simulink model "lorenz3d"  (Simulink 3.00)
settings: Solver=ode45  SolverMode=SingleTasking  StartTime=0.0  StopTime=inf  RelTol=1e-3  AbsTol=1e-6
undefined symbols (not defined in the file or in its folder): sfunxyz
settings Model: ExternalInput=[]  SaveTime=off  SaveOutput=off  InitialState=[]  IntegerOverflowMsg=none  RTWOptions="-aEnforceIntegerDowncast=1 -aFoldNonRolledExpr=1 -aInlineInvariantSignals=1 -aInlineParameters=0 -aLocalBlockOutputs=1 -aRollThreshold=5 -aZeroInternalMemoryAtStartup=1 -aZeroExternalMemoryAtStartup=1 -aInitFltsAndDblsToZero=1 -aGenerateReport=0 -aGenCodeOnly=0 -aRTWVerbose=1 -aIncludeHyperlinkInReport=0 -aLaunchReport=0 -aForceParamTrailComments=0 -aGenerateComments=1 -aIgnoreCustomStorageClasses=1 -aIncHierarchyInIds=0 -aMaxRTWIdLen=31 -aShowEliminatedStatements=0 -aPrefixModelToSubsysFcnNames=1 -aIncDataTypeInIds=0 -aInsertBlockDesc=0 -aSimulinkBlockComments=1 -aInlinedPrmAccess=\"Literals\"  -aSuppressErrorStatus=0 -aModelReferenceCompliant=1 -aSupportNonInlinedSFcns=1 -aSupportContinuousTime=1 -aSupportComplex=1 -aSupportNonFinite=1 -aSupportAbsoluteTime=1 -aTargetFcnLib=\"ansi_tfl_tmw.mat\" -aMultiInstanceERTCode=0 -aLogVarNameModifier=\"rt_\" -aIsPILTarget=0 -aCombineOutputUpdateFcns=0 -aGenerateASAP2=0 -aGenerateSampleERTMain=0 -aGenerateFullHeader=1 -aUtilityFuncGeneration=\"Auto\" -aIncludeFileDelimiter=\"Auto\" -aIncludeMdlTerminateFcn=1 -aPurelyIntegerCode=0 -aERTCustomFileBanners=0 -aRTWCAPIStates=0 -aRTWCAPIParams=0 -aRTWCAPISignals=0 -aMatFileLogging=1 -aGenFloatMathFcnCalls=\"ANSI_C\" -aExtModeMexFile=\"ext_comm\" -aExtModeTransport=0 -aExtModeStaticAllocSize=1000000 -aExtModeTesting=0 -aExtModeStaticAlloc=0 -aExtMode=0  -aInitFltsAndDblsToZero=1"  Creator=The MathWorks Inc.  LastModifiedBy=campa

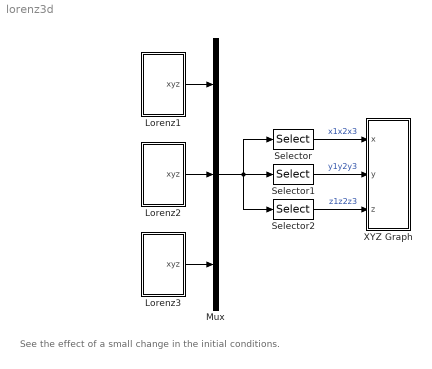
== system lorenz3d ==
  note: See the effect of a small change in the initial conditions.
  Lorenz1 : Subsystem  mask(Lorenz Attractor System){s=10, r=28, b=2+2/3, xyz0=[1 1 1]}
      mask prompts: s "sigma"; r "rho"; b "beta"; xyz0 "Initial State (x0, y0, y0)"
      mask help:
      | This autonomous system generates the lorentz attractor:
      | xdot=sigma*(x-y); ydot=rho*x-y-x*z; zdot=-beta*z+x*y;
      | Parameters and initial state can be selected from the mask.
      mask Help:
      | This autonomous system generates the lorentz attractor.
      | Parameters and initial state can be selected from the mask.
      | <p>
      | The system equations are:
      | xdot = sigma*(x-y),
      | ydot = rho*x-y-x*z,
      | zdot = -beta*z+x*y,
  Lorenz2 : Subsystem  mask(Lorenz Attractor System){s=10, r=28, b=2+2/3, xyz0=[2 2 2]}
      mask prompts: s "sigma"; r "rho"; b "beta"; xyz0 "Initial State (x0, y0, y0)"
      mask help:
      | This autonomous system generates the lorentz attractor:
      | xdot=sigma*(x-y); ydot=rho*x-y-x*z; zdot=-beta*z+x*y;
      | Parameters and initial state can be selected from the mask.
      mask Help:
      | This autonomous system generates the lorentz attractor.
      | Parameters and initial state can be selected from the mask.
      | <p>
      | The system equations are:
      | xdot = sigma*(x-y),
      | ydot = rho*x-y-x*z,
      | zdot = -beta*z+x*y,
  Lorenz3 : Subsystem  mask(Lorenz Attractor System){s=10, r=28, b=2+2/3, xyz0=[3 3 3]}
      mask prompts: s "sigma"; r "rho"; b "beta"; xyz0 "Initial State (x0, y0, y0)"
      mask help:
      | This autonomous system generates the lorentz attractor:
      | xdot=sigma*(x-y); ydot=rho*x-y-x*z; zdot=-beta*z+x*y;
      | Parameters and initial state can be selected from the mask.
      mask Help:
      | This autonomous system generates the lorentz attractor.
      | Parameters and initial state can be selected from the mask.
      | <p>
      | The system equations are:
      | xdot = sigma*(x-y),
      | ydot = rho*x-y-x*z,
      | zdot = -beta*z+x*y,
  Mux : Mux  Inputs=[3 3 3]
  Selector : Selector  Elements=[1 4 7]  InputPortWidth=9
  Selector1 : Selector  Elements=[2 5 8]  InputPortWidth=9
  Selector2 : Selector  Elements=[3 6 9]  InputPortWidth=9
  XYZ Graph : Subsystem  LoadFcn=sfunxyz([],[],[],'LoadBlock')  StartFcn=sfunxyz([],[],[],'Start')  StopFcn=sfunxyz([],[],[],'Stop')  mask(XYZ multiscope){np=3, xlim=[-30 30], ylim=[-20 30], zlim=[0 50], cp=[1 1 20], gd=on, st=0.01}
      mask prompts: np "Number of lines"; xlim "[xmin xmax]"; ylim "[ymin ymax]"; zlim "[zmin zmax]"; cp "Camera position (use [0 0 1] for 2D XY view)"; gd "Grid"; st "Sample time:"
      mask help:
      | Multidimensional XYZ scope using MATLAB graph window.
      |    X,Y,Z coordinates are respectively the first,second, and third input.
      |    Enter the number of lines, the XYZ ranges, the camera position,
      |    and the sampling time, as mask parameters.
      settings: CopyFcn=sfunxyz([],[],[],'CopyBlock')  DeleteFcn=sfunxyz([],[],[],'DeleteBlock')  NameChangeFcn=sfunxyz([],[],[],'NameChange')
      mask Help:
      | This block can be used to explore limit cycles.
      |    Look at the m-file sfunxyz.m to see how it works.
      mask Display: plot([.05 .95 .95 .05 .05],[.45 .45 .95 .95 .45], 0.5+cos(0:0.1:2*pi)*0.3,0.7+sin(0:0.1:2*pi)*0.2)
  wires:
  Lorenz1/1(xyz) -> Mux/1
  Lorenz2/1(xyz) -> Mux/2
  Mux/1 -> Selector/1, Selector1/1, Selector2/1
  Lorenz3/1(xyz) -> Mux/3
  Selector/1 -> XYZ Graph/1(x)  "x1x2x3"
  Selector1/1 -> XYZ Graph/2(y)  "y1y2y3"
  Selector2/1 -> XYZ Graph/3(z)  "z1z2z3"

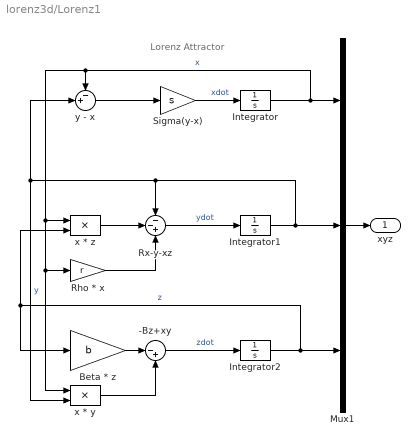
== system lorenz3d/Lorenz1 ==
  note: Lorenz Attractor
  -Bz+xy : Sum  Inputs=|-+  SaturateOnIntegerOverflow=on
  Beta * z : Gain  Gain=b  SaturateOnIntegerOverflow=on
  Integrator : Integrator  ExternalReset=none  InitialConditionSource=internal  InitialCondition=xyz0(1)  LimitOutput=off  UpperSaturationLimit=inf  LowerSaturationLimit=-inf  ShowSaturationPort=off  ShowStatePort=off  AbsoluteTolerance=auto
  Integrator1 : Integrator  ExternalReset=none  InitialConditionSource=internal  InitialCondition=xyz0(2)  LimitOutput=off  UpperSaturationLimit=inf  LowerSaturationLimit=-inf  ShowSaturationPort=off  ShowStatePort=off  AbsoluteTolerance=auto
  Integrator2 : Integrator  ExternalReset=none  InitialConditionSource=internal  InitialCondition=xyz0(3)  LimitOutput=off  UpperSaturationLimit=inf  LowerSaturationLimit=-inf  ShowSaturationPort=off  ShowStatePort=off  AbsoluteTolerance=auto
  Mux1 : Mux  Inputs=3
  Rho * x : Gain  Gain=r  SaturateOnIntegerOverflow=on
  Rx-y-xz : Sum  Inputs=--+  SaturateOnIntegerOverflow=on
  Sigma(y-x) : Gain  Gain=s  SaturateOnIntegerOverflow=on
  x * y : Product  Inputs=2  SaturateOnIntegerOverflow=on
  x * z : Product  Inputs=2  SaturateOnIntegerOverflow=on
  y - x : Sum  Inputs=-+|  SaturateOnIntegerOverflow=on
  xyz : Outport  Port=1
  wires:
  Sigma(y-x)/1 -> Integrator/1  "xdot"
  y - x/1 -> Sigma(y-x)/1
  Rx-y-xz/1 -> Integrator1/1  "ydot"
  x * z/1 -> Rx-y-xz/2
  Integrator2/1 -> x * z/2, Beta * z/1, Mux1/3  "z"
  Integrator1/1 -> Rx-y-xz/1, y - x/2, x * y/2, Mux1/2  "y"
  Integrator/1 -> y - x/1, x * z/1, Rho * x/1, x * y/1, Mux1/1  "x"
  -Bz+xy/1 -> Integrator2/1  "zdot"
  Beta * z/1 -> -Bz+xy/1
  x * y/1 -> -Bz+xy/2
  Mux1/1 -> xyz/1
  Rho * x/1 -> Rx-y-xz/3

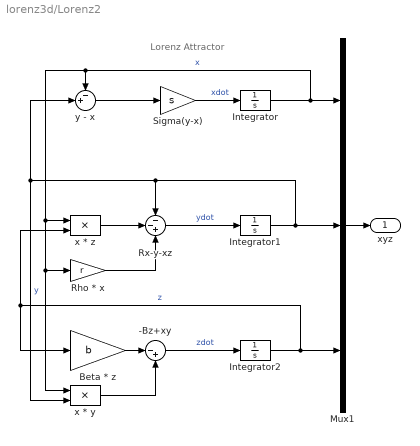
== system lorenz3d/Lorenz2 ==
  note: Lorenz Attractor
  -Bz+xy : Sum  Inputs=|-+  SaturateOnIntegerOverflow=on
  Beta * z : Gain  Gain=b  SaturateOnIntegerOverflow=on
  Integrator : Integrator  ExternalReset=none  InitialConditionSource=internal  InitialCondition=xyz0(1)  LimitOutput=off  UpperSaturationLimit=inf  LowerSaturationLimit=-inf  ShowSaturationPort=off  ShowStatePort=off  AbsoluteTolerance=auto
  Integrator1 : Integrator  ExternalReset=none  InitialConditionSource=internal  InitialCondition=xyz0(2)  LimitOutput=off  UpperSaturationLimit=inf  LowerSaturationLimit=-inf  ShowSaturationPort=off  ShowStatePort=off  AbsoluteTolerance=auto
  Integrator2 : Integrator  ExternalReset=none  InitialConditionSource=internal  InitialCondition=xyz0(3)  LimitOutput=off  UpperSaturationLimit=inf  LowerSaturationLimit=-inf  ShowSaturationPort=off  ShowStatePort=off  AbsoluteTolerance=auto
  Mux1 : Mux  Inputs=3
  Rho * x : Gain  Gain=r  SaturateOnIntegerOverflow=on
  Rx-y-xz : Sum  Inputs=--+  SaturateOnIntegerOverflow=on
  Sigma(y-x) : Gain  Gain=s  SaturateOnIntegerOverflow=on
  x * y : Product  Inputs=2  SaturateOnIntegerOverflow=on
  x * z : Product  Inputs=2  SaturateOnIntegerOverflow=on
  y - x : Sum  Inputs=-+|  SaturateOnIntegerOverflow=on
  xyz : Outport  Port=1
  wires:
  Mux1/1 -> xyz/1
  x * y/1 -> -Bz+xy/2
  Beta * z/1 -> -Bz+xy/1
  -Bz+xy/1 -> Integrator2/1  "zdot"
  Integrator/1 -> Mux1/1, x * y/1, Rho * x/1, x * z/1, y - x/1  "x"
  Integrator1/1 -> Mux1/2, x * y/2, y - x/2, Rx-y-xz/1  "y"
  Integrator2/1 -> Mux1/3, Beta * z/1, x * z/2  "z"
  x * z/1 -> Rx-y-xz/2
  Rx-y-xz/1 -> Integrator1/1  "ydot"
  y - x/1 -> Sigma(y-x)/1
  Sigma(y-x)/1 -> Integrator/1  "xdot"
  Rho * x/1 -> Rx-y-xz/3

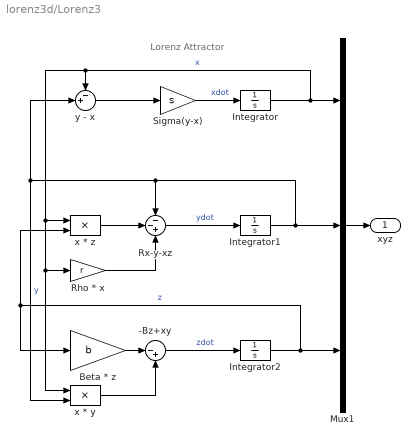
== system lorenz3d/Lorenz3 ==
  note: Lorenz Attractor
  -Bz+xy : Sum  Inputs=|-+  SaturateOnIntegerOverflow=on
  Beta * z : Gain  Gain=b  SaturateOnIntegerOverflow=on
  Integrator : Integrator  ExternalReset=none  InitialConditionSource=internal  InitialCondition=xyz0(1)  LimitOutput=off  UpperSaturationLimit=inf  LowerSaturationLimit=-inf  ShowSaturationPort=off  ShowStatePort=off  AbsoluteTolerance=auto
  Integrator1 : Integrator  ExternalReset=none  InitialConditionSource=internal  InitialCondition=xyz0(2)  LimitOutput=off  UpperSaturationLimit=inf  LowerSaturationLimit=-inf  ShowSaturationPort=off  ShowStatePort=off  AbsoluteTolerance=auto
  Integrator2 : Integrator  ExternalReset=none  InitialConditionSource=internal  InitialCondition=xyz0(3)  LimitOutput=off  UpperSaturationLimit=inf  LowerSaturationLimit=-inf  ShowSaturationPort=off  ShowStatePort=off  AbsoluteTolerance=auto
  Mux1 : Mux  Inputs=3
  Rho * x : Gain  Gain=r  SaturateOnIntegerOverflow=on
  Rx-y-xz : Sum  Inputs=--+  SaturateOnIntegerOverflow=on
  Sigma(y-x) : Gain  Gain=s  SaturateOnIntegerOverflow=on
  x * y : Product  Inputs=2  SaturateOnIntegerOverflow=on
  x * z : Product  Inputs=2  SaturateOnIntegerOverflow=on
  y - x : Sum  Inputs=-+|  SaturateOnIntegerOverflow=on
  xyz : Outport  Port=1
  wires:
  Sigma(y-x)/1 -> Integrator/1  "xdot"
  y - x/1 -> Sigma(y-x)/1
  Rx-y-xz/1 -> Integrator1/1  "ydot"
  x * z/1 -> Rx-y-xz/2
  Integrator2/1 -> x * z/2, Beta * z/1, Mux1/3  "z"
  Integrator1/1 -> Rx-y-xz/1, y - x/2, x * y/2, Mux1/2  "y"
  Integrator/1 -> y - x/1, x * z/1, Rho * x/1, x * y/1, Mux1/1  "x"
  -Bz+xy/1 -> Integrator2/1  "zdot"
  Beta * z/1 -> -Bz+xy/1
  x * y/1 -> -Bz+xy/2
  Mux1/1 -> xyz/1
  Rho * x/1 -> Rx-y-xz/3

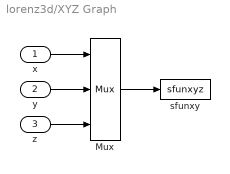
== system lorenz3d/XYZ Graph ==
  x : Inport  Port=1  PortWidth=-1  SampleTime=-1  DataType=auto
      settings: SignalType=auto
  y : Inport  Port=2  PortWidth=-1  SampleTime=-1  DataType=auto
      settings: SignalType=auto
  z : Inport  Port=3  PortWidth=-1  SampleTime=-1  DataType=auto
      settings: SignalType=auto
  Mux : Mux  Inputs=[np np np]
      settings: DisplayOption=none
  sfunxy : S-Function  FunctionName=sfunxyz  Parameters=[xlim ylim zlim],st,np,cp,gd  PortCounts=[]  SFunctionModules=''
  wires:
  Mux/1 -> sfunxy/1
  x/1 -> Mux/1
  y/1 -> Mux/2
  z/1 -> Mux/3
